simulink model "NewWatch"  (R2015a)
settings: Solver=ode3  StartTime=0.0  StopTime=inf  FixedStep=0.1  RelTol=1e-3
libraries: simulink x1
settings Model: CovSFcnEnable=off  Creator=Lorenzo  LastModifiedBy=Matteo
settings OptimizationCC: InlineParams=on  InlineInvariantSignals=on  OptimizeModelRefInitCode=on  LifeSpan=Inf
settings DebuggingCC: SolverPrmCheckMsg=warning
settings RTWCC: SystemTargetFile=ert.tlc  GenCodeOnly=on  TemplateMakefile=ert_default_tmf  Description=Embedded Coder
settings CodeAppCC: IgnoreCustomStorageClasses=off
settings ERTTargetCC: ParMdlRefBuildCompliant=on  CompOptLevelCompliant=on  ConcurrentExecutionCompliant=on  IncludeMdlTerminateFcn=off  ERTFirstTimeCompliant=on  SupportAbsoluteTime=off  MultiInstanceERTCode=on  CodeInterfacePackaging=Reusable function  SupportNonFinite=off  SupportComplex=off  PurelyIntegerCode=on  SupportContinuousTime=off  SupportVariableSizeSignals=off  ModelStepFunctionPrototypeControlCompliant=on  CPPClassGenCompliant=on  InlinedParameterPlacement=Hierarchical  MultiInstanceErrorCode=None  ERTCustomFileTemplate=example_file_process.tlc

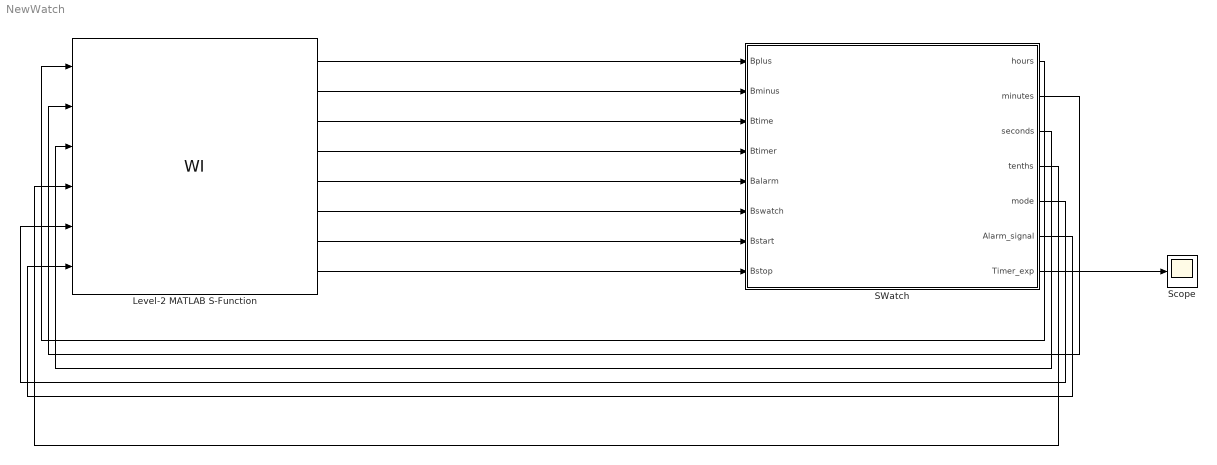
== system NewWatch ==
  Level-2 MATLAB S-Function : M-S-Function  FunctionName=WI
  SWatch : Subsystem
  Scope : Scope
  wires:
  Level-2 MATLAB S-Function/1 -> SWatch/1(Bplus)
  Level-2 MATLAB S-Function/2 -> SWatch/2(Bminus)
  Level-2 MATLAB S-Function/3 -> SWatch/3(Btime)
  Level-2 MATLAB S-Function/4 -> SWatch/4(Btimer)
  Level-2 MATLAB S-Function/5 -> SWatch/5(Balarm)
  Level-2 MATLAB S-Function/6 -> SWatch/6(Bswatch)
  SWatch/1(hours) -> Level-2 MATLAB S-Function/1
  SWatch/2(minutes) -> Level-2 MATLAB S-Function/2
  SWatch/3(seconds) -> Level-2 MATLAB S-Function/3
  SWatch/4(tenths) -> Level-2 MATLAB S-Function/4
  SWatch/5(mode) -> Level-2 MATLAB S-Function/5
  Level-2 MATLAB S-Function/7 -> SWatch/7(Bstart)
  Level-2 MATLAB S-Function/8 -> SWatch/8(Bstop)
  SWatch/6(Alarm_signal) -> Level-2 MATLAB S-Function/6
  SWatch/7(Timer_exp) -> Scope/1

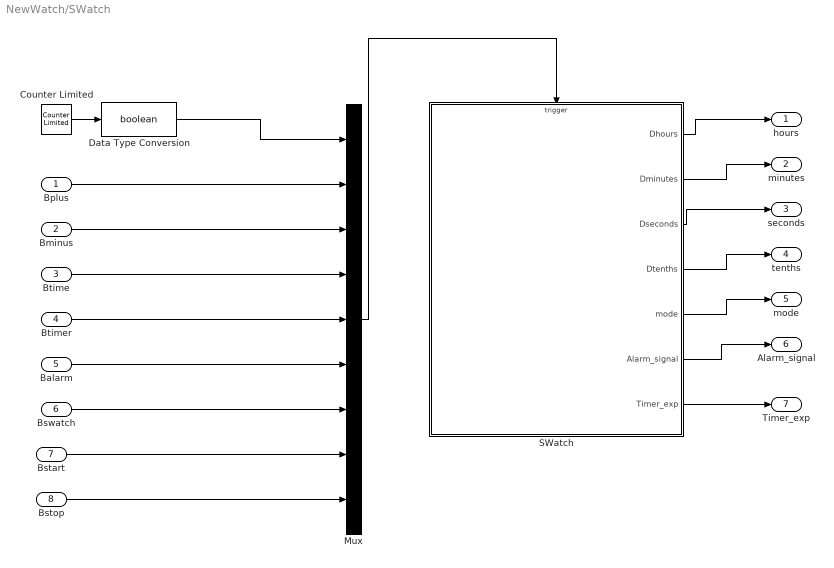
== system NewWatch/SWatch ==
  Bplus : Inport
  Bminus : Inport  Port=2
  Btime : Inport  Port=3
  Btimer : Inport  Port=4
  Balarm : Inport  Port=5
  Bswatch : Inport  Port=6
  Bstart : Inport  Port=7
  Bstop : Inport  Port=8  OutDataTypeStr=boolean
  Counter Limited : simulink/Sources/Counter Limited  uplimit=1  tsamp=0.1
  Data Type Conversion : DataTypeConversion  OutDataTypeStr=boolean
  Mux : Mux  Inputs=9
  SWatch : Stateflow chart  TreatAsAtomicUnit=on
  hours : Outport
  minutes : Outport  Port=2
  seconds : Outport  Port=3
  tenths : Outport  Port=4
  mode : Outport  Port=5
  Alarm_signal : Outport  Port=6
  Timer_exp : Outport  Port=7
  wires:
  SWatch/5(mode) -> mode/1
  SWatch/4(Dtenths) -> tenths/1
  SWatch/3(Dseconds) -> seconds/1
  Bminus/1 -> Mux/3
  Btime/1 -> Mux/4
  Data Type Conversion/1 -> Mux/1
  SWatch/2(Dminutes) -> minutes/1
  SWatch/1(Dhours) -> hours/1
  Bplus/1 -> Mux/2
  Bswatch/1 -> Mux/7
  Mux/1 -> SWatch/Trigger
  Balarm/1 -> Mux/6
  Counter Limited/1 -> Data Type Conversion/1
  Btimer/1 -> Mux/5
  Bstart/1 -> Mux/8
  Bstop/1 -> Mux/9
  SWatch/6(Alarm_signal) -> Alarm_signal/1
  SWatch/7(Timer_exp) -> Timer_exp/1

== stateflow chart NewWatch/SWatch/SWatch ==
  settings: executeAtInitialization=1
  state AlarmMng [parallel]
    settings: executionOrder=3
    state Alarm_signaler
    (default) -> Alarm_signaler : /{Alarm_signal= uint8(0);Alarm_h= uint8(0);Alarm_m= uint8(0);Alarm_state= uint8(0);}
    Alarm_signaler -> Alarm_signaler : [ptick && hours==Alarm_h && minutes == Alarm_m && Alarm_state == 1 && seconds == 0 && tenths ==0] {Alarm_signal= uint8(1); Alarm_state= uint8(0);}
  state Control [parallel]
    settings: executionOrder=1
    state timemode
      en: mode=uint8(0)
      timemode -> timemode [order 1] : ptick{Dhours=hours;Dminutes=minutes;Dseconds=seconds;Dtenths=tenths;}
    state timermode
      entry:mode=uint8(1)
      state setminutes
        en:Dminutes=Aminutes
      state sethours
        en:Dhours=Ahours;
      state setseconds
        en:Dseconds=Aseconds
      state Timer
        state Timer_Finish
          en:Timer_exp= uint8(1);
        state Timer_Start
        (default) -> Timer_Start
        (junction 302) -> Timer_Finish [order 4] : [Ahours==0 && Aminutes==0 && Aseconds==0]
        (junction 171) -> (junction 302) [order 1] : [Atenths==0]
        (junction 302) -> (junction 167) [order 3] : [Ahours>0 && Aminutes==0 && Aseconds==0]/{Ahours=Ahours-1;Dhours=Ahours;Aminutes= uint8(59);Dminutes= uint8(59);Aseconds= uint8(59);Dseconds= uint8(59);}
        (junction 302) -> (junction 167) [order 2] : [Aminutes>0 && Aseconds==0] / {Aminutes=Aminutes -1;Dminutes=Aminutes;Aseconds= uint8(59);Dseconds=Aseconds; }
        Timer_Start -> (junction 171) : ptick {Atenths = mod(Atenths+1,10);}
        (junction 302) -> (junction 167) [order 1] : [Aseconds>0]/{Aseconds=Aseconds-1;Dseconds=Aseconds;}
        (junction 171) -> (junction 167) [order 2]
        (junction 167) -> Timer_Start
      setseconds -> Control.timermode.sethours [order 1] : Btimer
      Control.timermode.setminutes -> Control.timermode.setminutes [order 3] : Bminus[Aminutes==0]/{Aminutes= uint8(59)}
      Control.timermode.sethours -> Control.timermode.sethours [order 3] : Bminus[Ahours==0]/{Ahours= uint8(23)}
      setseconds -> setseconds [order 3] : Bminus[Aseconds==0]/{Aseconds= uint8(59)}
      timermode -> Control.timermode.sethours [order 1] : [Bstop]/{Aseconds= uint8(0);Ahours= uint8(0);
          | Aminutes= uint8(0);Dhours=Ahours;
          | Dminutes=Aminutes;Dseconds=Aseconds;
          | Timer_exp= uint8(0);}
      Control.timermode.sethours -> Control.timermode.sethours [order 4] : Bminus/{Ahours=Ahours-1}
      Control.timermode.sethours -> Control.timermode.setminutes [order 1] : Btimer
      (default) -> Control.timermode.sethours : /{Aminutes= uint8(0);Ahours = uint8(0);
          | Aseconds= uint8(0);Atenths= uint8(0);
          |  Dminutes=Aminutes; Dhours=Ahours;Dseconds=Aseconds;}
      Control.timermode.setminutes -> Control.timermode.setminutes [order 4] : Bminus/{Aminutes=Aminutes-1}
      Control.timermode.setminutes -> setseconds [order 1] : Btimer
      setseconds -> setseconds [order 4] : Bminus/{Aseconds=Aseconds-1}
      Control.timermode.sethours -> Timer [order 5] : Bstart[Ahours>0 || Aminutes>0 || Aseconds >0]
      Control.timermode.setminutes -> Control.timermode.setminutes [order 2] : Bplus/{Aminutes=mod(Aminutes+1,60)}
      Control.timermode.setminutes -> Timer [order 5] : Bstart[Ahours>0 || Aminutes>0 || Aseconds>0]
      Control.timermode.sethours -> Control.timermode.sethours [order 2] : Bplus/{Ahours=mod(Ahours+1,24)}
      setseconds -> Timer [order 5] : Bstart[Ahours>0 || Aminutes>0 || Aseconds >0]
      setseconds -> setseconds [order 2] : Bplus/{Aseconds=mod(Aseconds+1,60)}
    state Timeset
      state setminutes
        en:Dminutes=minutes
      state sethours
        en:
        Dhours=hours
      Control.Timeset.setminutes -> Control.Timeset.setminutes [order 3] : Bminus[minutes==0]/{minutes= uint8(59)}
      Control.Timeset.setminutes -> Control.Timeset.setminutes [order 4] : [Bminus]/{minutes=minutes-1}
      Control.Timeset.sethours -> Control.Timeset.setminutes [order 1] : [Btime]
      Control.Timeset.setminutes -> Control.Timeset.setminutes [order 2] : [Bplus]/{minutes=mod(minutes+1,60)}
      Control.Timeset.setminutes -> Control.Timeset.sethours [order 1] : [Btime]
      Control.Timeset.sethours -> Control.Timeset.sethours [order 3] : Bminus[hours==0]/{hours= uint8(23)}
      Control.Timeset.sethours -> Control.Timeset.sethours [order 4] : [Bminus]/{hours=hours-1}
      (default) -> Control.Timeset.sethours
      Control.Timeset.sethours -> Control.Timeset.sethours [order 2] : [Bplus]/{hours=mod(hours+1,24)}
    state swatchmode
      en:mode=uint8(3)
      state stop
        entry:
        Dhours=Ahours;
        Dminutes=Aminutes;
        Dseconds=Aseconds;
        Dtenths=Atenths;
      state start
        entry:
        Dhours=Ahours;
        Dminutes=Aminutes;
        Dseconds=Aseconds;
        Dtenths=Atenths;
      (default) -> stop : /{Ahours=uint8(0);Aminutes=uint8(0);Aseconds=uint8(0);Atenths=uint8(0);}
      start -> (junction 216) [order 3] : ptick/{Atenths = mod(Atenths+1,10);}
      (junction 216) -> (junction 228) [order 2]
      (junction 216) -> (junction 224) [order 1] : [Atenths==0]{Aseconds=mod(Aseconds+1,60);}
      stop -> start [order 1] : Bstart
      (junction 228) -> start
      (junction 224) -> (junction 228) [order 2]
      (junction 221) -> (junction 228) [order 2]
      (junction 224) -> (junction 221) [order 1] : [Aseconds==0]{Aminutes=mod(Aminutes+1,60);}
      start -> stop [order 1] : Bstop
      start -> stop [order 2] : Bswatch/{Ahours= uint8(0);
          | Aminutes= uint8(0);
          | Aseconds= uint8(0);
          | Atenths= uint8(0);}
      (junction 223) -> start
      stop -> stop [order 2] : Bswatch/{Ahours= uint8(0);
          | Aminutes= uint8(0);
          | Aseconds= uint8(0);
          | Atenths= uint8(0);}
      (junction 221) -> (junction 223) [order 1] : [Aminutes==0]{Ahours=mod(Ahours+1,24);}
    state alarmmode
      en:mode=uint8(2)
      state setminutes
        en:Dminutes=Aminutes
      state sethours
        en:Dhours=Ahours
      (default) -> Control.alarmmode.sethours : /{Aminutes= uint8(0);Ahours= uint8(0);Dhours=Ahours;Dminutes=Aminutes;Alarm_state= uint8(0);}
      Control.alarmmode.setminutes -> Control.alarmmode.setminutes [order 3] : Bminus[Aminutes==0]/{Aminutes= uint8(59)}
      Control.alarmmode.sethours -> Control.alarmmode.sethours [order 3] : Bminus[Ahours==0]/{Ahours= uint8(23)}
      Control.alarmmode.sethours -> Control.alarmmode.sethours [order 4] : Bminus/{Ahours=Ahours-1}
      Control.alarmmode.setminutes -> Control.alarmmode.setminutes [order 4] : Bminus/{Aminutes=Aminutes-1}
      Control.alarmmode.sethours -> Control.alarmmode.setminutes [order 1] : Balarm
      Control.alarmmode.setminutes -> Control.alarmmode.setminutes [order 5] : Bstart/ {Alarm_state= uint8(1);
          | Alarm_h=Ahours;
          | Alarm_m=Aminutes;}
      Control.alarmmode.sethours -> Control.alarmmode.sethours [order 5] : Bstart/ {Alarm_state= uint8(1);Alarm_h=Ahours;Alarm_m=Aminutes;}
      Control.alarmmode.setminutes -> Control.alarmmode.sethours [order 1] : Balarm
      Control.alarmmode.sethours -> Control.alarmmode.sethours [order 2] : Bplus/{Ahours=mod(Ahours+1,24)}
      Control.alarmmode.setminutes -> Control.alarmmode.setminutes [order 2] : Bplus/{Aminutes=mod(Aminutes+1,60)}
      alarmmode -> alarmmode [order 1] : Bstop /{Alarm_signal= uint8(0);}
    timermode -> timemode [order 3] : Btime
    (default) -> timemode : {Ahours= uint8(0); Aminutes= uint8(0);Aseconds= uint8(0);Atenths= uint8(0);}
    timemode -> timermode [order 1] : Btimer
    timemode -> Timeset [order 4] : Btime / {hours= uint8(0);seconds= uint8(0);minutes= uint8(0);tenths= uint8(0);mutex= uint8(1);Dseconds= uint8(0);Dminutes= uint8(0);Dtenths= uint8(0)}
    timermode -> timemode [order 4] : Btime
    swatchmode -> timermode [order 1] : Btimer
    Timeset -> timemode : Bstart/{mutex= uint8(0)}
    timermode -> swatchmode [order 2] : Bswatch
    alarmmode -> timermode [order 1] : Btimer
    timermode -> alarmmode [order 1] : Balarm
    timemode -> alarmmode [order 2] : Balarm
    timemode -> swatchmode [order 3] : Bswatch
    swatchmode -> timemode [order 3] : Btime
    alarmmode -> timemode [order 3] : Btime
    swatchmode -> alarmmode [order 2] : Balarm
    alarmmode -> swatchmode [order 2] : Bswatch
  state TimeCount [parallel]
    settings: executionOrder=2
    state timecount
    (default) -> timecount : /{hours=uint8(0);minutes=uint8(0);seconds=uint8(0);tenths=uint8(0); mutex = uint8(0);}
    timecount -> (junction 19) : [ptick && mutex==0] {tenths = mod(tenths+1,10);}
    (junction 32) -> timecount
    (junction 34) -> timecount
    (junction 19) -> (junction 34) [order 2]
    (junction 19) -> (junction 27) [order 1] : [tenths==0]{seconds=mod(seconds+1,60);}
    (junction 27) -> (junction 34) [order 2]
    (junction 27) -> (junction 30) [order 1] : [seconds==0]{minutes=mod(minutes+1,60);}
    (junction 30) -> (junction 34) [order 2]
    (junction 30) -> (junction 32) [order 1] : [minutes==0]{hours=mod(hours+1,24);}
  data: hours local uint8; minutes local uint8; seconds local uint8; tenths local uint8; Dhours output uint8; Dminutes output uint8; Dseconds output uint8; Dtenths output uint8; mode output uint8; Ahours local uint8; Aminutes local uint8; Aseconds local uint8; Atenths local uint8; Alarm_h local uint8; Alarm_m local uint8; Alarm_state local uint8; Alarm_signal output uint8; mutex local uint8; Timer_exp output uint8
  events: ptick input EITHER_EDGE_EVENT; Bplus input RISING_EDGE_EVENT; Bminus input RISING_EDGE_EVENT; Btime input RISING_EDGE_EVENT; Btimer input RISING_EDGE_EVENT; Balarm input RISING_EDGE_EVENT; Bswatch input RISING_EDGE_EVENT; Bstart input RISING_EDGE_EVENT; Bstop input RISING_EDGE_EVENT
